simulink model "Simulation_model"  (R2020b)
settings: Solver=VariableStepAuto  StartTime=0.0  StopTime=15  MaxStep=1e-4  RelTol=1e-3
values from neighbouring files (symbols this model uses):
  Ga = 3    [Exam_202007.m]    (also in Levitator.m = 0.4; Problem_P1.m = 0.095; Problem_P1me.m = 0.095; Problem_P2.m = -0.09)
  Gf = 1/(Kd*Gs)    (= 0.2)    [Exam_202007.m]    (also in Levitator.m = 1; Problem_P1.m = 1; Problem_P1me.m = 1; Problem_P2.m = 1)
  Gs = 5    [Exam_202007.m]    (also in Levitator.m = 555.89; Problem_P1.m = 1; Problem_P1me.m = 1; Problem_P2.m = 1)
  Kd = 1    [Exam_202007.m]    (also in Levitator.m = 0.00179891705193; Problem_P1.m; Problem_P2.m; Problem_P3.m)
libraries: cstblocks x2, simulink x2
settings Model: Creator=Diego Regruto  LastModifiedBy=kevin
settings SFSimCC: CustomCodeUndefinedFunction=UseInterfaceOnly

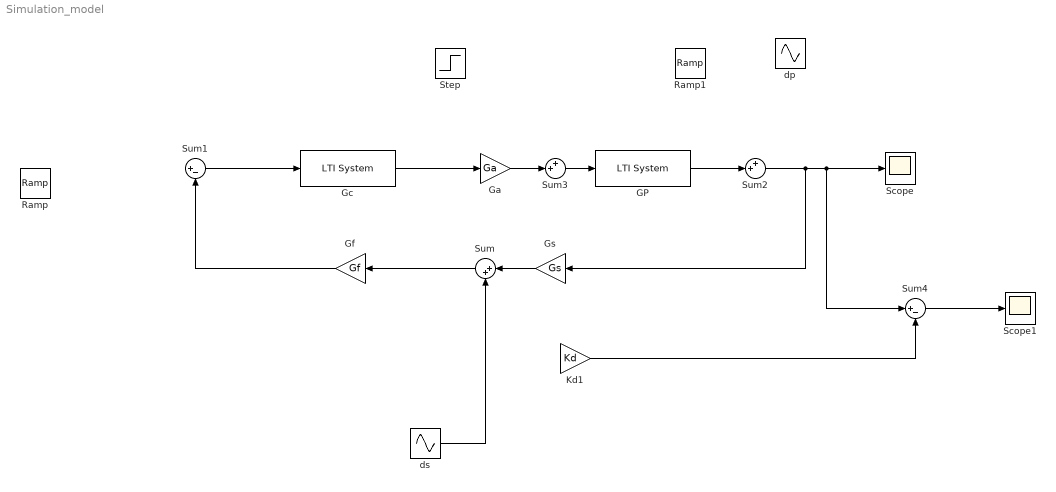
== system Simulation_model ==
  GP : cstblocks/LTI System  sys=Gp  IC=[]
  Ga : Gain  Gain=Ga
  Gc : cstblocks/LTI System  sys=Gc  IC=[]
  Gf : Gain  Gain=Gf
  Gs : Gain  Gain=Gs
  Kd1 : Gain  Gain=Kd
  Ramp : simulink/Sources/Ramp  slope=1  start=0  InitialOutput=0
  Ramp1 : simulink/Sources/Ramp  slope=3e-3  start=0  InitialOutput=0
  Scope : Scope
  Scope1 : Scope
  Step : Step  Time=0  After=8.5e-3  SampleTime=0
  Sum : Sum  Inputs=|++
  Sum1 : Sum  Inputs=|+-
  Sum2 : Sum  Inputs=++|
  Sum3 : Sum  Inputs=++|
  Sum4 : Sum  Inputs=|+-
  dp : Sin  Amplitude=2e-2  Frequency=0.02  SampleTime=0
  ds : Sin  Amplitude=10^-2  Frequency=50  SampleTime=0
  wires:
  Gc/1 -> Ga/1
  Sum/1 -> Gf/1
  Gs/1 -> Sum/1
  Sum1/1 -> Gc/1
  Gf/1 -> Sum1/2
  GP/1 -> Sum2/2
  Sum2/1 -> Sum4/1, Scope/1, Gs/1
  Sum3/1 -> GP/1
  Ga/1 -> Sum3/2
  Kd1/1 -> Sum4/2
  Sum4/1 -> Scope1/1
  ds/1 -> Sum/2
